simulink model "Modelo"  (R2022b)
settings: Solver=ode45  StartTime=0.0  StopTime=5  MaxStep=1e-5  MinStep=1e-12  RelTol=1e-3
values from neighbouring files (symbols this model uses):
  A = theta(:,1:end-1)    [EstimacionLeon.m]
  B = (theta(:,end))    [EstimacionLeon.m]
settings Model: Creator=unam-  LastModifiedBy=unam-

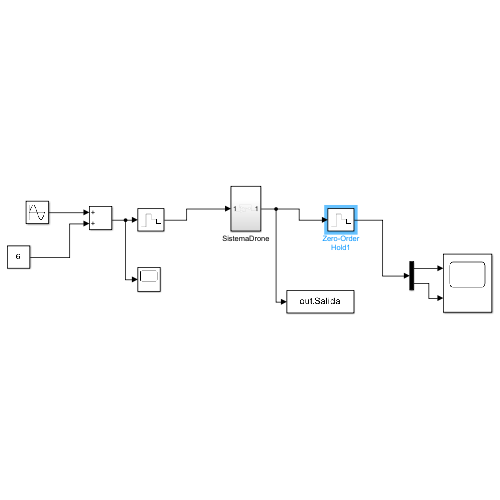
[thumbnail: Simulink's stored preview of the top-level diagram]
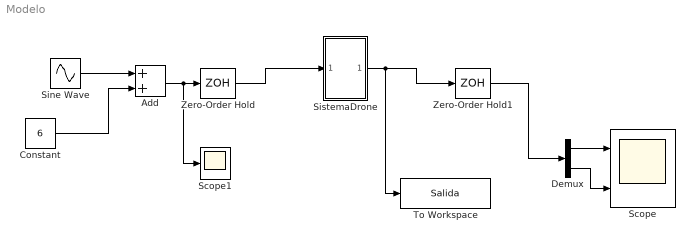
== system Modelo ==
  Add : Sum
  Constant : Constant  Value=6
  Demux : Demux  Outputs=2
  Scope : Scope  NumInputPorts=2
  Scope1 : Scope
  Sine Wave : Sin  Amplitude=6  Frequency=2*pi  SampleTime=0
  SistemaDrone : Subsystem
  To Workspace : ToWorkspace  VariableName=Salida  SaveFormat=Timeseries  SampleTime=-1
  Zero-Order Hold : ZeroOrderHold  SampleTime=1e-3
  Zero-Order Hold1 : ZeroOrderHold  SampleTime=1e-3
  wires:
  SistemaDrone/1(Out1) -> To Workspace/1, Zero-Order Hold1/1
  Zero-Order Hold/1 -> SistemaDrone/1(In1)
  Demux/1 -> Scope/1
  Demux/2 -> Scope/2
  Zero-Order Hold1/1 -> Demux/1
  Add/1 -> Scope1/1, Zero-Order Hold/1
  Sine Wave/1 -> Add/1
  Constant/1 -> Add/2

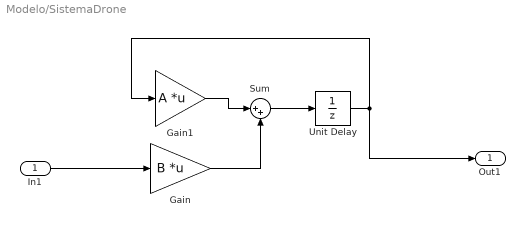
== system Modelo/SistemaDrone ==
  In1 : Inport
  Gain : Gain  Gain=B  Multiplication=Matrix(K*u)
  Gain1 : Gain  Gain=A  Multiplication=Matrix(K*u)
  Sum : Sum  Inputs=|++
  Unit Delay : UnitDelay  SampleTime=1e-3  HasFrameUpgradeWarning=on
  Out1 : Outport
  wires:
  Unit Delay/1 -> Out1/1, Gain1/1
  Sum/1 -> Unit Delay/1
  Gain/1 -> Sum/2
  In1/1 -> Gain/1
  Gain1/1 -> Sum/1
